simulink model "Pong2D"  (Simulink 8.6)
settings: Solver=ode4  StartTime=0.0  StopTime=inf  FixedStep=0.001  RelTol=1e-3
undefined symbols (not defined in the file or in its folder): damping, lateral_damping, M_ball, stiffness, Visualization
libraries: quarc_library x9, simulink x3
settings Model: Creator=RSamra  LastModifiedBy=Mech430  SimulationMode=external  ExtModeTrigDuration=5000
settings SolverCC: PositivePriorityOrder=on
settings OptimizationCC: InitFltsAndDblsToZero=on
settings DebuggingCC: FcnCallInpInsideContextMsg=UseLocalSettings
settings SFSimCC: SimParseCustomCode=off
settings RTWCC: SystemTargetFile=quarc_win64.tlc  TemplateMakefile=quarc_default_tmf  Description=QUARC Win64 Target
settings STFCustomTargetCC: TargetPreCompLibLocation=C:\PROGRA~3\QUARC\lib\2015b\win64\release  ConcurrentExecutionCompliant=on  GeneratePreprocessorConditionals=Disable all  CombineOutputUpdateFcns=on  CPPClassGenCompliant=on  GRTInterface=off  SystemTargetFile=quarc_win64.tlc
settings GRTTargetCC: TargetPreCompLibLocation=C:\PROGRA~3\QUARC\lib\2015b\win64\release  ParMdlRefBuildCompliant=off  CompOptLevelCompliant=off  CombineOutputUpdateFcns=on  MatFileLogging=off  GRTInterface=off  UseToolchainInfoCompliant=off  ExtMode=on  ExtModeMexFile=quarc_comm

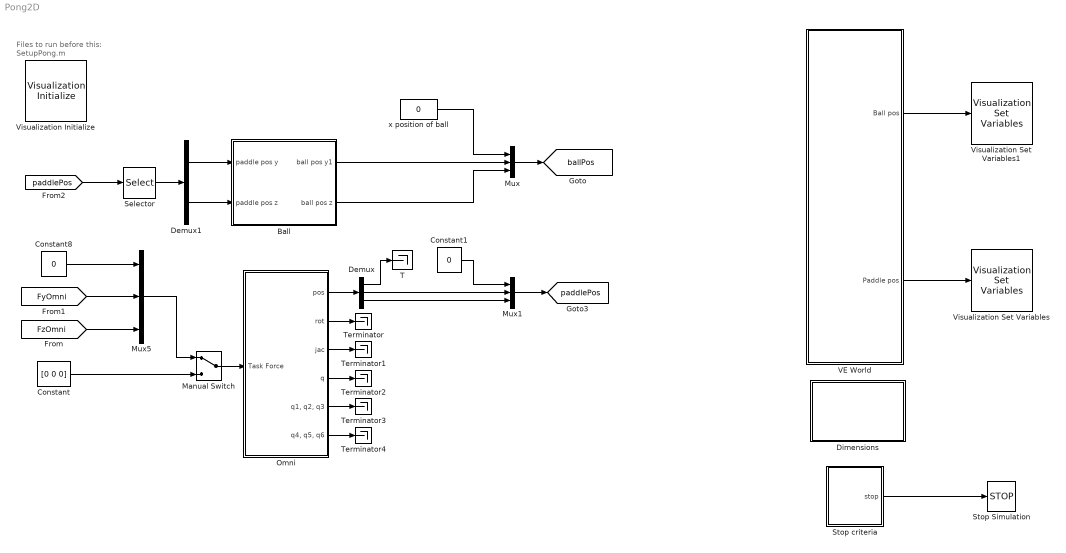
== system Pong2D ==
  note: Files to run before this:
      | SetupPong.m
  Ball : Subsystem
  Constant : Constant  Value=[0 0 0]
  Constant1 : Constant  Value=0  VectorParams1D=off  SampleTime=0
  Constant8 : Constant  Value=0  VectorParams1D=off  SampleTime=0
  Demux : Demux  Outputs=3
  Demux1 : Demux  Outputs=2
  Dimensions : Subsystem
  Manual Switch : ManualSwitch
  Mux : Mux  Inputs=3
  Mux1 : Mux  Inputs=3
  Mux5 : Mux  Inputs=3
  Omni : Subsystem
  Selector : Selector  InputPortWidth=3  IndexOptions=Index vector (dialog)  Indices=[2 3]  OutputSizes=1
  Stop Simulation : Stop
  Stop criteria : Subsystem
  T : Terminator
  Terminator{,1..4} (5 alike) : Terminator
  VE World : Subsystem
  Visualization Initialize : quarc_library/User Interface/Visualization/Visualization Initialize  object_name=Visualization-1  scene_file=Visualization\Haptic_Pong.xml  uri={'normal','';'Configuration','shmem://%m:2';}  apply_uri_to_all_configs=off  server_send_size=1000000  server_receive_size=1000  derive_from_server=on  client_send_size=1000  client_receive_size=1000000  variables=[ 40 60 ]  initial_values=single([ 0 0 -0.5 0 0 0 ])  open_on_start=on  close_on_stop=on
      settings: AttributesFormatString=%<object_name>
  Visualization Set Variables : quarc_library/User Interface/Visualization/Visualization Set Variables  object_name=Visualization-1  offset=[ 0 ]  data_type=[ 0 ]  length=[ 3 ]  sample_time=visualization_get_frame_period  actor_name={'actor.paddle/Position'}
      settings: AttributesFormatString=(%<object_name>)
  Visualization Set Variables1 : quarc_library/User Interface/Visualization/Visualization Set Variables  object_name=Visualization-1  offset=[ 3 ]  data_type=[ 0 ]  length=[ 3 ]  sample_time=visualization_get_frame_period  actor_name={'actor.ball/Position'}
      settings: AttributesFormatString=(%<object_name>)
  x position of ball : Constant  Value=0  VectorParams1D=off  SampleTime=0
  tag scope: ballPos=global, paddlePos=global
  wires:
  Mux/1 -> [ballPos]
  Stop criteria/1(stop) -> Stop Simulation/1
  x position of ball/1 -> Mux/1
  Constant1/1 -> Mux1/1
  Mux1/1 -> [paddlePos]
  Omni/1(pos) -> Demux/1
  Demux/1 -> T/1
  Constant/1 -> Manual Switch/2
  Manual Switch/1 -> Omni/1(Task Force)
  Constant8/1 -> Mux5/1
  Mux5/1 -> Manual Switch/1
  [FzOmni] -> Mux5/3
  Demux/2 -> Mux1/2
  Demux/3 -> Mux1/3
  Ball/1(ball pos y1) -> Mux/2
  Ball/2(ball pos z) -> Mux/3
  VE World/2(Paddle pos) -> Visualization Set Variables/1
  VE World/1(Ball pos) -> Visualization Set Variables1/1
  Omni/2(rot) -> Terminator/1
  Omni/3(jac) -> Terminator1/1
  Omni/4(q) -> Terminator2/1
  Omni/5("q1, q2, q3") -> Terminator3/1
  Omni/6("q4, q5, q6") -> Terminator4/1
  [paddlePos] -> Selector/1
  Selector/1 -> Demux1/1
  [FyOmni] -> Mux5/2
  Demux1/1 -> Ball/1(paddle pos y)
  Demux1/2 -> Ball/2(paddle pos z)

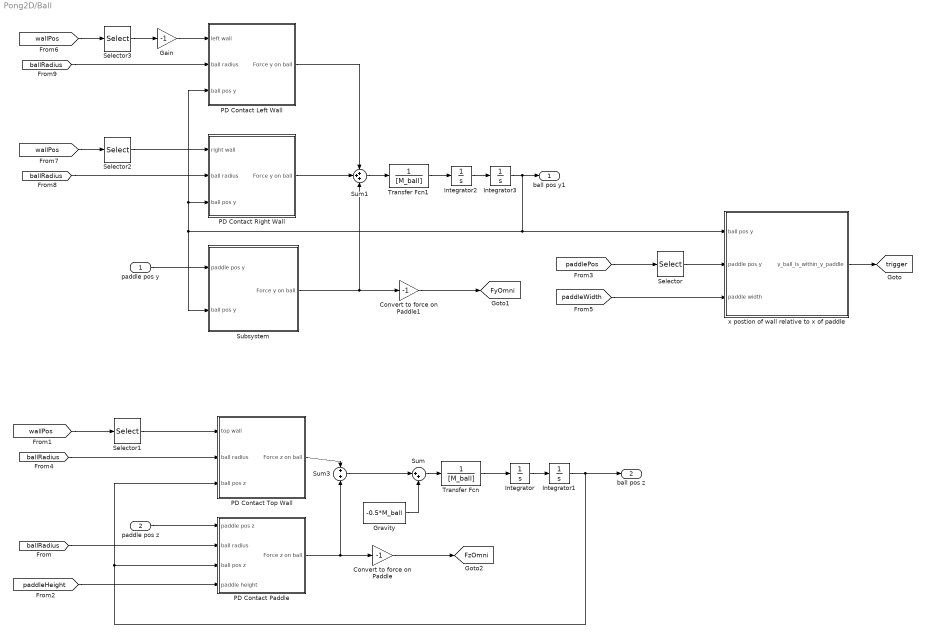
== system Pong2D/Ball ==
  paddle pos y : Inport
  paddle pos z : Inport  Port=2
  Convert to force on Paddle : Gain  Gain=-1
  Convert to force on Paddle1 : Gain  Gain=-1
  Gain : Gain  Gain=-1
  Gravity : Constant  Value=-0.5*M_ball  SampleTime=0
  Integrator{,1..3} (4 alike) : Integrator
  PD Contact Left Wall : Subsystem
  PD Contact Paddle : Subsystem
  PD Contact Right Wall : Subsystem
  PD Contact Top Wall : Subsystem
  Selector : Selector  InputPortWidth=3  IndexOptions=Index vector (dialog)  Indices=2  OutputSizes=1
  Selector1 : Selector  InputPortWidth=3  IndexOptions=Index vector (dialog)  Indices=3  OutputSizes=1
  Selector2 : Selector  InputPortWidth=3  IndexOptions=Index vector (dialog)  Indices=2  OutputSizes=1
  Selector3 : Selector  InputPortWidth=3  IndexOptions=Index vector (dialog)  Indices=2  OutputSizes=1
  Subsystem : Subsystem
  Sum : Sum  Inputs=|++
  Sum1 : Sum  Inputs=+++
  Sum3 : Sum
  Transfer Fcn : TransferFcn  Denominator=[M_ball]
  Transfer Fcn1 : TransferFcn  Denominator=[M_ball]
  x postion of wall relative to x of paddle : Subsystem
  ball pos y1 : Outport
  ball pos z : Outport  Port=2
  tag scope: FyOmni=global, FzOmni=global, trigger=global
  wires:
  Transfer Fcn/1 -> Integrator/1
  Integrator/1 -> Integrator1/1
  Sum/1 -> Transfer Fcn/1
  Gravity/1 -> Sum/2
  Integrator1/1 -> ball pos z/1, PD Contact Top Wall/3(ball pos z), PD Contact Paddle/3(ball pos z)
  PD Contact Top Wall/1("Force z on ball ") -> Sum3/1
  PD Contact Paddle/1(Force z on ball) -> Sum3/2, Convert to force on Paddle/1
  Sum3/1 -> Sum/1
  Convert to force on Paddle/1 -> [FzOmni]
  [ballRadius] -> PD Contact Top Wall/2(ball radius)
  paddle pos z/1 -> PD Contact Paddle/1(paddle pos z)
  [paddleHeight] -> PD Contact Paddle/4(paddle height)
  [ballRadius] -> PD Contact Paddle/2(ball radius)
  Selector1/1 -> PD Contact Top Wall/1(top wall)
  [wallPos] -> Selector1/1
  [paddleWidth] -> x postion of wall relative to x of paddle/3(paddle width)
  x postion of wall relative to x of paddle/1(y_ball_is_within_y_paddle) -> [trigger]
  Integrator3/1 -> ball pos y1/1, x postion of wall relative to x of paddle/1(ball pos y), Subsystem/2(ball pos y), PD Contact Left Wall/3(ball pos y), PD Contact Right Wall/3(ball pos y)
  [paddlePos] -> Selector/1
  Selector/1 -> x postion of wall relative to x of paddle/2(paddle pos y)
  [wallPos] -> Selector2/1
  [wallPos] -> Selector3/1
  Selector3/1 -> Gain/1
  [ballRadius] -> PD Contact Left Wall/2(ball radius)
  [ballRadius] -> PD Contact Right Wall/2(ball radius)
  PD Contact Left Wall/1("Force y on ball ") -> Sum1/1
  PD Contact Right Wall/1("Force y on ball ") -> Sum1/2
  Transfer Fcn1/1 -> Integrator2/1
  Integrator2/1 -> Integrator3/1
  Sum1/1 -> Transfer Fcn1/1
  paddle pos y/1 -> Subsystem/1(paddle pos y)
  Subsystem/1(Force y on ball) -> Convert to force on Paddle1/1, Sum1/3
  Convert to force on Paddle1/1 -> [FyOmni]
  Gain/1 -> PD Contact Left Wall/1(left wall)
  Selector2/1 -> PD Contact Right Wall/1(right wall)

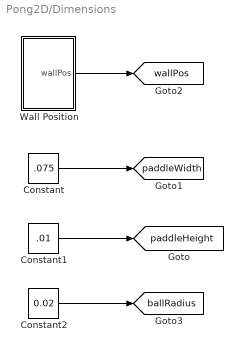
== system Pong2D/Dimensions ==
  Constant : Constant  Value=.075  VectorParams1D=off  SampleTime=0
  Constant1 : Constant  Value=.01  VectorParams1D=off  SampleTime=0
  Constant2 : Constant  Value=0.02  VectorParams1D=off
  Wall Position : Subsystem
  tag scope: ballRadius=global, paddleHeight=global, paddleWidth=global, wallPos=global
  wires:
  Constant/1 -> [paddleWidth]
  Constant2/1 -> [ballRadius]
  Constant1/1 -> [paddleHeight]
  Wall Position/1(wallPos) -> [wallPos]

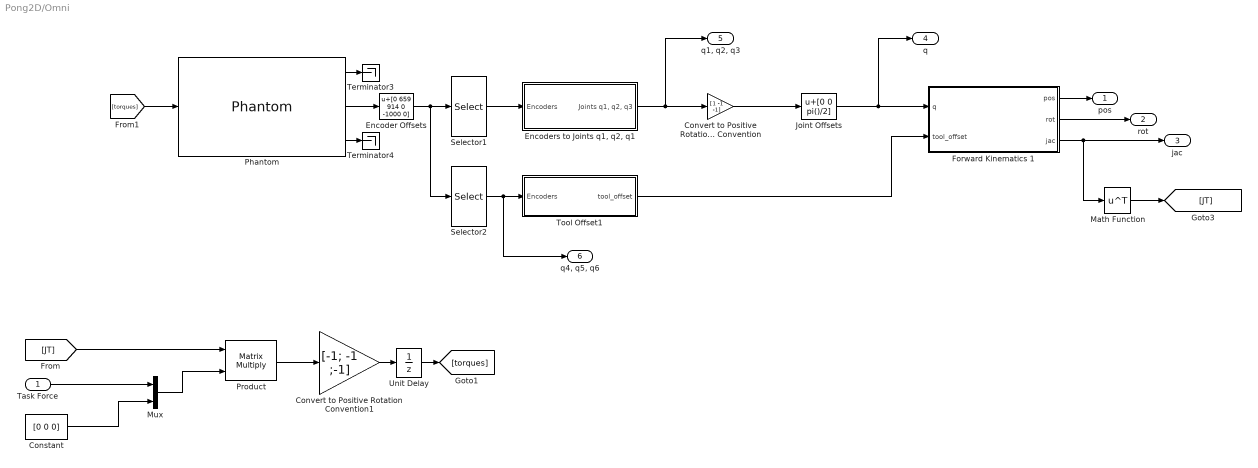
== system Pong2D/Omni ==
  Task Force : Inport
  Constant : Constant  Value=[0 0 0]
  Convert to Positive Rotation Convention : Gain  Gain=[1 -1 -1]
  Convert to Positive Rotation Convention1 : Gain  Gain=[-1; -1 ;-1]
  Encoder Offsets : Bias  Bias=[0 659 914 0 -1000 0]
  "Encoders to Joints q1, q2, q1" : Subsystem
  Forward Kinematics 1 : MATLAB Function  TreatAsAtomicUnit=on
  Joint Offsets : Bias  Bias=[0 0 pi()/2]
  Math Function : Math  Operator=transpose  SaturateOnIntegerOverflow=on
  Mux : Mux  Inputs=2
  Phantom : quarc_library/Devices/Third-Party/SensAble/Phantom/Phantom  device_name=Default Device  output_type=Encoders Values  input_type=Joint space  velocity_limit_option=on  velocity_limit=1200  is_7dof=off  sample_time=-1
      settings: AttributesFormatString=(%<device_name>)
  Product : Product  Multiplication=Matrix(*)  RndMeth=Zero
  Selector1 : Selector  InputPortWidth=6  IndexOptions=Index vector (dialog)  Indices=[1:3]  OutputSizes=1
  Selector2 : Selector  InputPortWidth=6  IndexOptions=Index vector (dialog)  Indices=[4:6]  OutputSizes=1
  Terminator3 : Terminator
  Terminator4 : Terminator
  Tool Offset1 : MATLAB Function  TreatAsAtomicUnit=on
  Unit Delay : UnitDelay  SampleTime=-1
  pos : Outport
  rot : Outport  Port=2
  jac : Outport  Port=3
  q : Outport  Port=4
  "q1, q2, q3" : Outport  Port=5
  "q4, q5, q6" : Outport  Port=6
  wires:
  Math Function/1 -> [JT]
  Forward Kinematics 1/3(jac) -> Math Function/1, jac/1
  [JT] -> Product/1
  Forward Kinematics 1/1(pos) -> pos/1
  Forward Kinematics 1/2(rot) -> rot/1
  Constant/1 -> Mux/2
  Task Force/1 -> Mux/1
  Mux/1 -> Product/2
  Convert to Positive Rotation Convention/1 -> Joint Offsets/1
  Convert to Positive Rotation Convention1/1 -> Unit Delay/1
  Joint Offsets/1 -> q/1, Forward Kinematics 1/1(q)
  Product/1 -> Convert to Positive Rotation Convention1/1
  Phantom/2 -> Encoder Offsets/1
  [torques] -> Phantom/1
  Phantom/3 -> Terminator4/1
  Phantom/1 -> Terminator3/1
  Selector2/1 -> Tool Offset1/1(Encoders), "q4, q5, q6"/1
  Selector1/1 -> "Encoders to Joints q1, q2, q1"/1(Encoders)
  Encoder Offsets/1 -> Selector1/1, Selector2/1
  "Encoders to Joints q1, q2, q1"/1("Joints q1, q2, q3") -> Convert to Positive Rotation Convention/1, "q1, q2, q3"/1
  Tool Offset1/1(tool_offset) -> Forward Kinematics 1/2(tool_offset)
  Unit Delay/1 -> [torques]

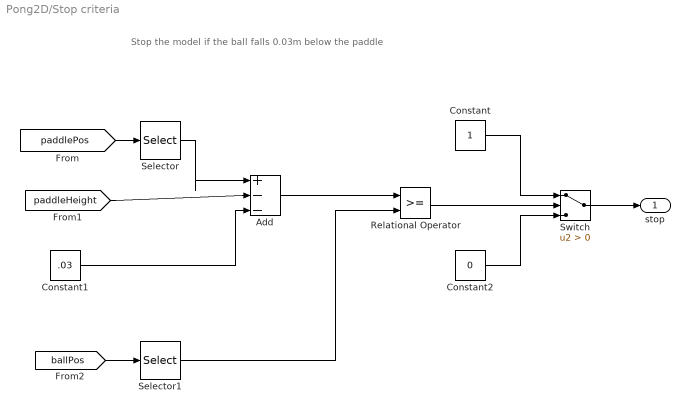
== system Pong2D/Stop criteria ==
  note: Stop the model if the ball falls 0.03m below the paddle
  Add : Sum  Inputs=|+--
  Constant : Constant  SampleTime=0
  Constant1 : Constant  Value=.03  SampleTime=0
  Constant2 : Constant  Value=0  SampleTime=0
  Relational Operator : RelationalOperator  OutDataTypeStr=boolean
  Selector : Selector  InputPortWidth=3  IndexOptions=Index vector (dialog)  Indices=3  OutputSizes=1
  Selector1 : Selector  InputPortWidth=3  IndexOptions=Index vector (dialog)  Indices=3  OutputSizes=1
  Switch : Switch  Criteria=u2 > Threshold
  stop : Outport
  wires:
  [paddleHeight] -> Add/2
  Add/1 -> Relational Operator/1
  Relational Operator/1 -> Switch/2
  Constant/1 -> Switch/1
  Constant2/1 -> Switch/3
  [paddlePos] -> Selector/1
  [ballPos] -> Selector1/1
  Constant1/1 -> Add/3
  Switch/1 -> stop/1
  Selector/1 -> Add/1
  Selector1/1 -> Relational Operator/2

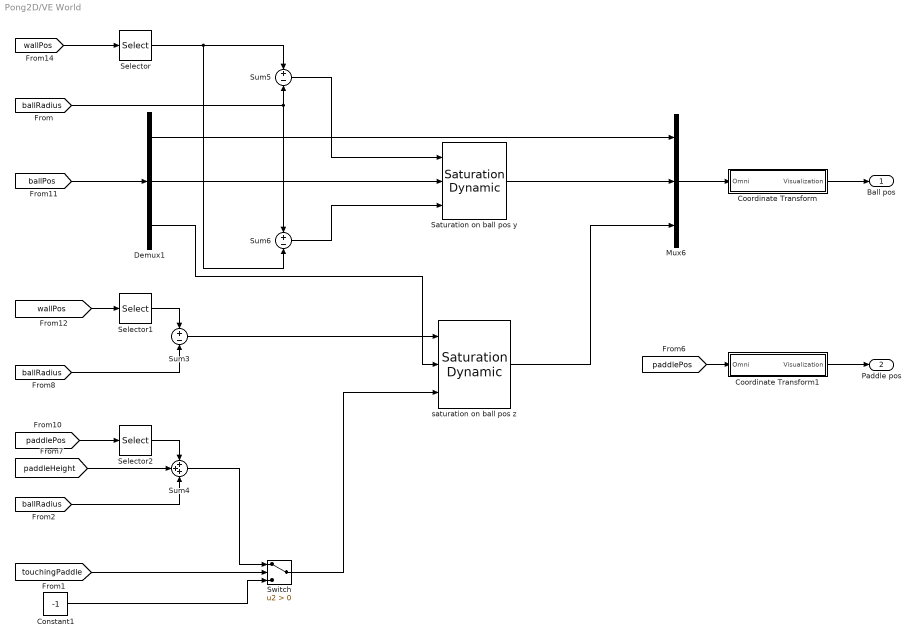
== system Pong2D/VE World ==
  Constant1 : Constant  Value=-1
  Coordinate Transform : Subsystem
  Coordinate Transform1 : Subsystem
  Demux1 : Demux  Outputs=3
  Mux6 : Mux  Inputs=3
  Saturation on ball pos y : simulink/Discontinuities/Saturation Dynamic  OutMin=[]  OutMax=[]  OutDataTypeStr=Inherit: Same as second input  OutDataType=sfix(16)  OutScaling=2^-10  DoSatur=off
  Selector : Selector  InputPortWidth=3  IndexOptions=Index vector (dialog)  Indices=2  OutputSizes=1
  Selector1 : Selector  InputPortWidth=3  IndexOptions=Index vector (dialog)  Indices=3  OutputSizes=1
  Selector2 : Selector  InputPortWidth=3  IndexOptions=Index vector (dialog)  Indices=3  OutputSizes=1
  Sum3 : Sum  Inputs=+-
  Sum4 : Sum  Inputs=+++
  Sum5 : Sum  Inputs=+-
  Sum6 : Sum  Inputs=+-
  Switch : Switch  Criteria=u2 > Threshold
  saturation on ball pos z : simulink/Discontinuities/Saturation Dynamic  OutMin=[]  OutMax=[]  OutDataTypeStr=Inherit: Same as second input  OutDataType=sfix(16)  OutScaling=2^-10  DoSatur=off
  Ball pos : Outport
  Paddle pos : Outport  Port=2
  wires:
  [paddlePos] -> Coordinate Transform1/1(Omni)
  [ballPos] -> Demux1/1
  [wallPos] -> Selector1/1
  [paddlePos] -> Selector2/1
  [paddleHeight] -> Sum4/2
  [ballRadius] -> Sum4/3
  [ballRadius] -> Sum3/2
  [ballRadius] -> Sum5/2, Sum6/1
  Sum5/1 -> Saturation on ball pos y/1
  Mux6/1 -> Coordinate Transform/1(Omni)
  Sum6/1 -> Saturation on ball pos y/3
  Switch/1 -> saturation on ball pos z/3
  [touchingPaddle] -> Switch/2
  Sum4/1 -> Switch/1
  Constant1/1 -> Switch/3
  Sum3/1 -> saturation on ball pos z/1
  [wallPos] -> Selector/1
  Coordinate Transform1/1("Visualization ") -> Paddle pos/1
  Coordinate Transform/1("Visualization ") -> Ball pos/1
  Demux1/2 -> Saturation on ball pos y/2
  Demux1/3 -> saturation on ball pos z/2
  Demux1/1 -> Mux6/1
  Saturation on ball pos y/1 -> Mux6/2
  saturation on ball pos z/1 -> Mux6/3
  Selector/1 -> Sum5/1, Sum6/2
  Selector1/1 -> Sum3/1
  Selector2/1 -> Sum4/1

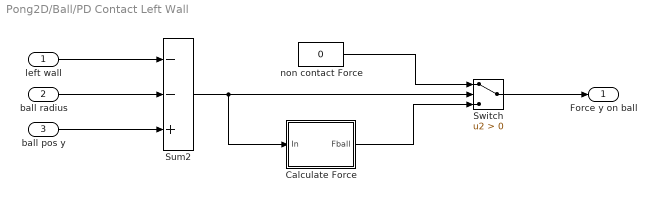
== system Pong2D/Ball/PD Contact Left Wall ==
  left wall : Inport
  ball radius : Inport  Port=2
  ball pos y : Inport  Port=3
  Calculate Force : Subsystem
  Sum2 : Sum  Inputs=--+
  Switch : Switch  Criteria=u2 > Threshold
  non contact Force : Constant  Value=0  VectorParams1D=off  SampleTime=0
  "Force y on ball " : Outport
  wires:
  Sum2/1 -> Calculate Force/1(In), Switch/2
  ball radius/1 -> Sum2/2
  left wall/1 -> Sum2/1
  Switch/1 -> "Force y on ball "/1
  ball pos y/1 -> Sum2/3
  non contact Force/1 -> Switch/1
  Calculate Force/1(Fball) -> Switch/3

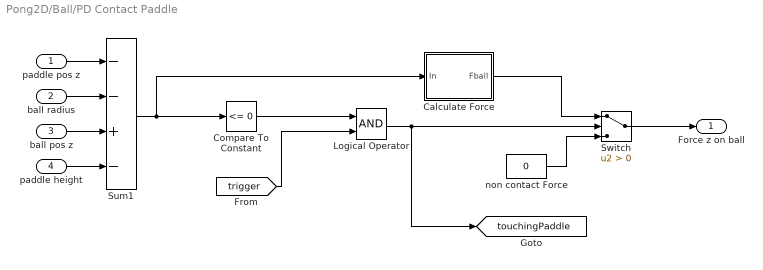
== system Pong2D/Ball/PD Contact Paddle ==
  paddle pos z : Inport
  ball radius : Inport  Port=2
  ball pos z : Inport  Port=3
  paddle height : Inport  Port=4
  Calculate Force : Subsystem
  Compare To Constant : simulink/Logic and Bit Operations/Compare To Constant  relop=<=  const=0  OutDataTypeStr=uint8  ZeroCross=off
  Logical Operator : Logic  AllPortsSameDT=off  OutDataTypeStr=boolean
  Sum1 : Sum  Inputs=--+-
  Switch : Switch  Criteria=u2 > Threshold
  non contact Force : Constant  Value=0  VectorParams1D=off  SampleTime=0
  Force z on ball : Outport
  tag scope: touchingPaddle=global
  wires:
  Sum1/1 -> Compare To Constant/1, Calculate Force/1(In)
  Compare To Constant/1 -> Logical Operator/1
  [trigger] -> Logical Operator/2
  Logical Operator/1 -> Switch/2, [touchingPaddle]
  paddle pos z/1 -> Sum1/1
  Switch/1 -> Force z on ball/1
  paddle height/1 -> Sum1/4
  Calculate Force/1(Fball) -> Switch/1
  non contact Force/1 -> Switch/3
  ball pos z/1 -> Sum1/3
  ball radius/1 -> Sum1/2

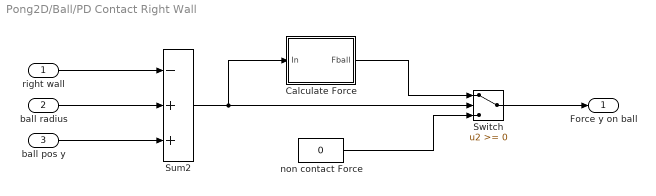
== system Pong2D/Ball/PD Contact Right Wall ==
  right wall : Inport
  ball radius : Inport  Port=2
  ball pos y : Inport  Port=3
  Calculate Force : Subsystem
  Sum2 : Sum  Inputs=-++
  Switch : Switch
  non contact Force : Constant  Value=0  VectorParams1D=off  SampleTime=0
  "Force y on ball " : Outport
  wires:
  ball pos y/1 -> Sum2/3
  Switch/1 -> "Force y on ball "/1
  right wall/1 -> Sum2/1
  ball radius/1 -> Sum2/2
  Sum2/1 -> Switch/2, Calculate Force/1(In)
  non contact Force/1 -> Switch/3
  Calculate Force/1(Fball) -> Switch/1

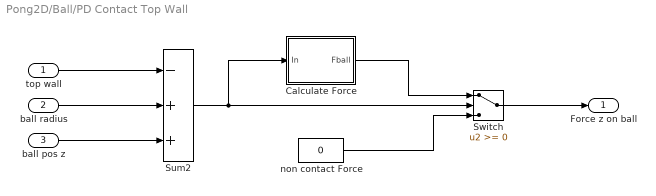
== system Pong2D/Ball/PD Contact Top Wall ==
  top wall : Inport
  ball radius : Inport  Port=2
  ball pos z : Inport  Port=3
  Calculate Force : Subsystem
  Sum2 : Sum  Inputs=-++
  Switch : Switch
  non contact Force : Constant  Value=0  VectorParams1D=off  SampleTime=0
  "Force z on ball " : Outport
  wires:
  ball pos z/1 -> Sum2/3
  Switch/1 -> "Force z on ball "/1
  top wall/1 -> Sum2/1
  ball radius/1 -> Sum2/2
  Sum2/1 -> Switch/2, Calculate Force/1(In)
  non contact Force/1 -> Switch/3
  Calculate Force/1(Fball) -> Switch/1

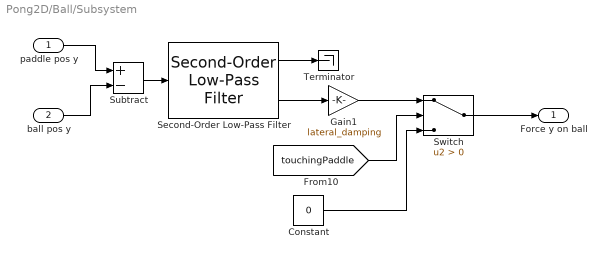
== system Pong2D/Ball/Subsystem ==
  paddle pos y : Inport
  ball pos y : Inport  Port=2
  Constant : Constant  Value=0
  Gain1 : Gain  Gain=lateral_damping
  Second-Order Low-Pass Filter : quarc_library/Continuous/Second-Order Low-Pass Filter  params_source=Internal (dialog parameters)  input_width=200  input_zeta=1  input_init=0
  Subtract : Sum  Inputs=+-
  Switch : Switch  Criteria=u2 > Threshold
  Terminator : Terminator
  Force y on ball : Outport
  wires:
  Second-Order Low-Pass Filter/2 -> Gain1/1
  Switch/1 -> Force y on ball/1
  [touchingPaddle] -> Switch/2
  Gain1/1 -> Switch/1
  ball pos y/1 -> Subtract/2
  Subtract/1 -> Second-Order Low-Pass Filter/1
  Second-Order Low-Pass Filter/1 -> Terminator/1
  paddle pos y/1 -> Subtract/1
  Constant/1 -> Switch/3

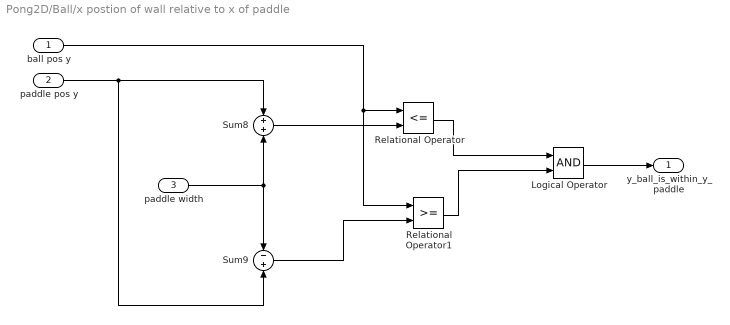
== system Pong2D/Ball/x postion of wall relative to x of paddle ==
  ball pos y : Inport
  paddle pos y : Inport  Port=2
  paddle width : Inport  Port=3
  Logical Operator : Logic  AllPortsSameDT=off  OutDataTypeStr=boolean
  Relational Operator : RelationalOperator  Operator=<=  OutDataTypeStr=boolean
  Relational Operator1 : RelationalOperator  OutDataTypeStr=boolean
  Sum8 : Sum
  Sum9 : Sum  Inputs=-+
  y_ball_is_within_y_paddle : Outport
  wires:
  Sum8/1 -> Relational Operator/2
  Sum9/1 -> Relational Operator1/2
  Relational Operator/1 -> Logical Operator/1
  Relational Operator1/1 -> Logical Operator/2
  ball pos y/1 -> Relational Operator/1, Relational Operator1/1
  paddle pos y/1 -> Sum8/1, Sum9/2
  paddle width/1 -> Sum8/2, Sum9/1
  Logical Operator/1 -> y_ball_is_within_y_paddle/1

== system Pong2D/Dimensions/Wall Position ==
  Add : Sum
  Constant : Constant  Value=[0 0 0.11]  VectorParams1D=off  SampleTime=0
  Constant1 : Constant  Value=0.2  SampleTime=0
  wallPos : Outport
  wires:
  Constant1/1 -> Add/1
  Constant/1 -> Add/2
  Add/1 -> wallPos/1

== system Pong2D/Omni/Encoders to Joints q1, q2, q1 ==
  Encoders : Inport
  Bias1 : Bias  Bias=[0 -659 -910]
  Embedded MATLAB Function : MATLAB Function  TreatAsAtomicUnit=on
  Encoder : Gain  Gain=2*pi/2048
  Gear Ratio : Gain  Gain=1./[7.461 -7.519 7.529]
  "Joints q1, q2, q3" : Outport
  wires:
  Embedded MATLAB Function/1(q) -> "Joints q1, q2, q3"/1
  Encoders/1 -> Bias1/1
  Encoder/1 -> Gear Ratio/1
  Gear Ratio/1 -> Embedded MATLAB Function/1(m)
  Bias1/1 -> Encoder/1

== system Pong2D/VE World/Coordinate Transform ==
  Omni : Inport
  Gain : Gain  Gain=[-10 -10 10]
  "Visualization " : Outport
  wires:
  Omni/1 -> Gain/1
  Gain/1 -> "Visualization "/1

== system Pong2D/VE World/Coordinate Transform1 ==
  Omni : Inport
  Gain : Gain  Gain=[-10 -10 10]
  "Visualization " : Outport
  wires:
  Gain/1 -> "Visualization "/1
  Omni/1 -> Gain/1

== system Pong2D/Ball/PD Contact Left Wall/Calculate Force ==
  In : Inport
  Convert to force on ball : Gain  Gain=-1
  Damping : Gain  Gain=damping
  Second-Order Low-Pass Filter : quarc_library/Continuous/Second-Order Low-Pass Filter  params_source=Internal (dialog parameters)  input_width=200  input_zeta=1  input_init=0
  Stiffness : Gain  Gain=stiffness
  Subtract : Sum
  Terminator : Terminator
  Fball : Outport
  wires:
  Second-Order Low-Pass Filter/1 -> Terminator/1
  Second-Order Low-Pass Filter/2 -> Damping/1
  Convert to force on ball/1 -> Fball/1
  Subtract/1 -> Convert to force on ball/1
  Damping/1 -> Subtract/2
  Stiffness/1 -> Subtract/1
  In/1 -> Second-Order Low-Pass Filter/1, Stiffness/1

== system Pong2D/Ball/PD Contact Paddle/Calculate Force ==
  In : Inport
  Convert to force on ball : Gain  Gain=-1
  Damping : Gain  Gain=damping
  Second-Order Low-Pass Filter : quarc_library/Continuous/Second-Order Low-Pass Filter  params_source=Internal (dialog parameters)  input_width=200  input_zeta=1  input_init=0
  Stiffness : Gain  Gain=stiffness
  Subtract : Sum
  Terminator : Terminator
  Fball : Outport
  wires:
  Subtract/1 -> Convert to force on ball/1
  Damping/1 -> Subtract/2
  Second-Order Low-Pass Filter/2 -> Damping/1
  Stiffness/1 -> Subtract/1
  In/1 -> Stiffness/1, Second-Order Low-Pass Filter/1
  Convert to force on ball/1 -> Fball/1
  Second-Order Low-Pass Filter/1 -> Terminator/1

== system Pong2D/Ball/PD Contact Right Wall/Calculate Force ==
  In : Inport
  Convert to force on ball : Gain  Gain=-1
  Damping : Gain  Gain=damping
  Second-Order Low-Pass Filter : quarc_library/Continuous/Second-Order Low-Pass Filter  params_source=Internal (dialog parameters)  input_width=200  input_zeta=1  input_init=0
  Stiffness : Gain  Gain=stiffness
  Subtract : Sum
  Terminator : Terminator
  Fball : Outport
  wires:
  In/1 -> Stiffness/1, Second-Order Low-Pass Filter/1
  Stiffness/1 -> Subtract/1
  Damping/1 -> Subtract/2
  Subtract/1 -> Convert to force on ball/1
  Convert to force on ball/1 -> Fball/1
  Second-Order Low-Pass Filter/2 -> Damping/1
  Second-Order Low-Pass Filter/1 -> Terminator/1

== system Pong2D/Ball/PD Contact Top Wall/Calculate Force ==
  In : Inport
  Convert to force on ball : Gain  Gain=-1
  Damping : Gain  Gain=damping
  Second-Order Low-Pass Filter : quarc_library/Continuous/Second-Order Low-Pass Filter  params_source=Internal (dialog parameters)  input_width=200  input_zeta=1  input_init=0
  Stiffness : Gain  Gain=stiffness
  Subtract : Sum
  Terminator : Terminator
  Fball : Outport
  wires:
  In/1 -> Stiffness/1, Second-Order Low-Pass Filter/1
  Stiffness/1 -> Subtract/1
  Damping/1 -> Subtract/2
  Subtract/1 -> Convert to force on ball/1
  Convert to force on ball/1 -> Fball/1
  Second-Order Low-Pass Filter/2 -> Damping/1
  Second-Order Low-Pass Filter/1 -> Terminator/1

== matlab function Omni/Forward Kinematics 1 ==
  data: pos output double; q input double; rot output double; tool_offset input double; jac output double
function [pos,rot,jac]    = ForwardKinematics(q,tool_offset)
% This block supports the Embedded MATLAB subset.
% See the help menu for details. 

% Link lengths
L1 = .132;
L2 = .132;

%Define A-matrices
%A1= DH(theta ,d ,a ,alpha)
A1 = DH(q(1), 0, 0, -pi()/2);
A2 = DH(q(2), 0, L1, 0);
A3 = DH(q(3)-pi/2, 0, L2, 0);

%Define T Matrices
T01=A1;
T02=T01*A2;
T03=T02*A3;

%tool_offset given with respect to frame 3.
T_tool=T03*tool_offset;
rot=T_tool(1:3,1:3);
pos=T_tool(1:3,4);

%Axes of rotation in base coordinates. 
z0=[0 0 1]';
z1=T01(1:3,3);
z2=T02(1:3,3);

%Coordinate Frame origins in Base frame coordinates
p0=[0 0 0]';
p1=T01(1:3,4);
p2=T02(1:3,4);
p3=T03(1:3,4);

%Formulation of the Jacobian

%%%%%%%%%%%%%%%%%%%%%%%%%%%%JACOBIAN%%%%%%%%%%%%%%%%%%%%%%%%
jac = [cross(z0,(pos-p0)) cross(z1,(pos-p1)) cross(z2,(pos-p2))
    z0 z1 z2];

end

function A = DH(theta, d, a, alpha)

A_R_z = [cos(theta) -sin(theta) 0 0;
         sin(theta) cos(theta) 0 0;
         0 0 1 0;
         0 0 0 1];

A_T_z = [1 0 0 0;
         0 1 0 0;
         0 0 1 d;
         0 0 0 1];
     
  

A_T_x = [1 0 0 a;
         0 1 0 0;
         0 0 1 0;
         0 0 0 1];

A_R_x = [1 0 0 0;
         0 cos(alpha) -sin(alpha)  0;
         0 sin(alpha) cos(alpha) 0;
         0 0 0 1];

A = A_R_z*A_T_z*A_T_x*A_R_x;

end

== matlab function Omni/Tool Offset1 ==
  data: Encoders input double; tool_offset output double
function tool_offset = getToolOffset(Encoders)

%convert encoder values to angles using bias and gain
bias = [-2048 -2654 -2048];
gain = [2*pi()/4915 2*pi()/4096 2*pi()/4915];
Angle = (Encoders' + bias).*gain;

% convert the angle to the positive rotation convention defined
% by DH parameters
pos_rot = [-1 1 1];
joint_offset = [0 -(40-180)*pi/180 0];
Joint456 = Angle.*pos_rot + joint_offset;

%pick off theta4 and theta5
theta4 = Joint456(1);
theta5 = Joint456(2);

% The orientation of the tool offset matrix is given two successive
% rotations about x and z axis. 
RotZ = [cos(theta5) -sin(theta5) 0; sin(theta5) cos(theta5) 0; 0 0 1];
RotX = [1 0 0; 0 cos(theta4) -sin(theta4); 0 sin(theta4) cos(theta4)];
R = RotX*RotZ; % R is the rotation matrix of the tool offset matrix with respect to frame 3

% with respect to frame 3, the tool is 0.039m in the x-direction. Convert
% this vector to tool frame coordinates
tool_pos =R * [.039; 0; 0];

%create a Tool_offset transformation matrix. Use Identity matrix for
%rotation to show that the end effector frame and frame 3 are always
%aligned
I = [1 0 0; 0 1 0; 0 0 1];
tool = cat(2,I,tool_pos);
tool_offset = cat(1,tool,[0 0 0 1]);

== matlab function Omni/Encoders to Joints q1, q2, q1/Embedded MATLAB Function ==
  data: m input double; q output double
function q = Motors_2_Joints(m)
q = m;
q(1) = m(1);
q(2) = m(2);
q(3) = m(3) - m(2) -pi/2;
end
